simulink library "lagrange"  (R2023a)
settings: Solver=VariableStepAuto  StartTime=0.0  StopTime=10.0  RelTol=1e-3
undefined symbols (not defined in the file): b, d, g, J1, J2, J3, L, m
settings Model: Creator=Alex  LastModifiedBy=Alex

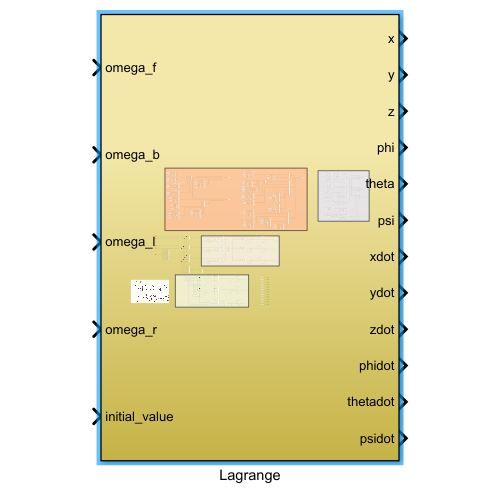
[thumbnail: Simulink's stored preview of the top-level diagram]
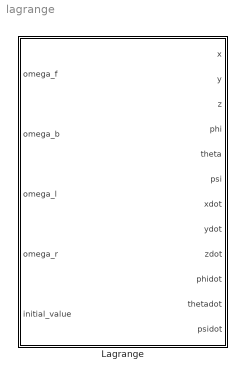
== system lagrange ==
  Lagrange : Subsystem

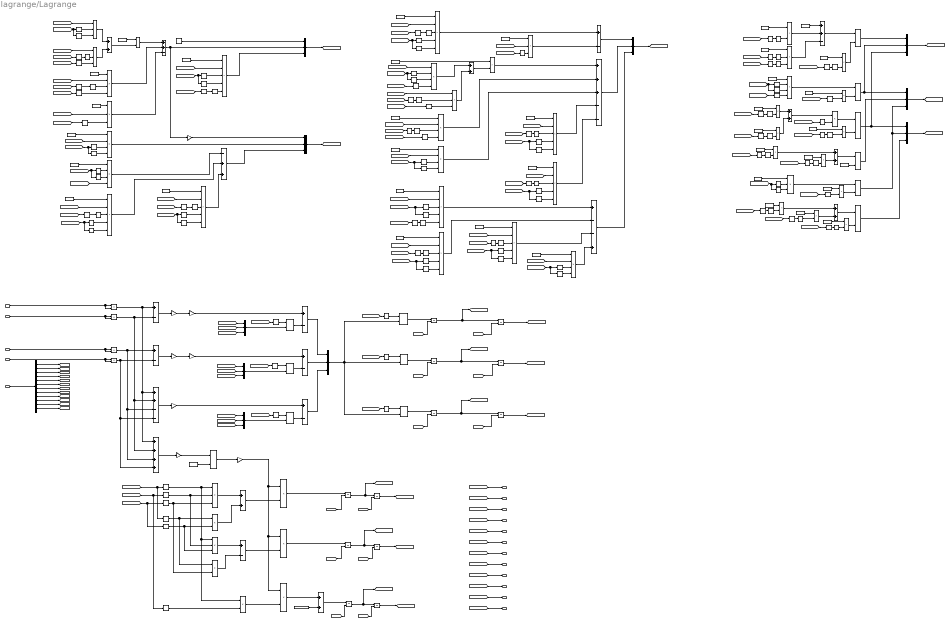
== system lagrange/Lagrange ==
  note: Rotational dynamics
  note: Matrix J^(-1) computation
  note: matrix C computation
  note: Translational dynamics
  omega_f : Inport
  omega_b : Inport  Port=2
  omega_l : Inport  Port=3
  omega_r : Inport  Port=4
  initial_value : Inport  Port=5
  Add{,1,8,11,14..16} (7 alike) : Sum  Inputs=+-
  Add{3,5,10,12,18..20} (7 alike) : Sum
  Add13 : Sum  Inputs=+--+
  Add17 : Sum  Inputs=++-
  Add2 : Sum  Inputs=++--
  Add4 : Sum  Inputs=++-
  Add6 : Sum  Inputs=++++
  Add7 : Sum  Inputs=-++
  Add9 : Sum  Inputs=+++--
  Constant : Constant  Value=0
  Constant{1,11,14,18} (4 alike) : Constant  Value=J2-J3
  Constant{10,17,20,30,33,38} (6 alike) : Constant  Value=J3
  Constant{4,8,12,15,21} (5 alike) : Constant  Value=J1
  Constant{2,5,7,13} (4 alike) : Constant  Value=J3-J2
  Constant{9,16,19,29,32,37} (6 alike) : Constant  Value=J2
  Constant{22,26,28,31,34,36} (6 alike) : Constant  Value=J2*J3
  Constant23 : Constant  Value=(J1-J3)*J2
  Constant24 : Constant  Value=(J2-J3)*J1
  Constant25 : Constant  Value=J1*J2*J3
  Constant27 : Constant  Value=-(J2-J3)
  Constant3 : Constant  Value=g
  Constant35 : Constant  Value=-(J2-J3)
  Constant6 : Constant  Value=m
  Cos{,1..7,9..10,12,15,17..18,20..21,23..24,28..30,32,34,36,38,40..41,44..45,47,49,53..55,58,60,63..64,66..67,69} (41 alike) : Trigonometry  Operator=cos
  Cos{8,11,13..14,16,19,22,25..27,31,33,35,37,39,42..43,46,48,50..52,56..57,59,61..62,65,68} (29 alike) : Trigonometry
  Demux : Demux  Outputs=12
  Divide{,1..6} (7 alike) : Product  Inputs=*/
  Gain : Gain  Gain=b
  Gain1 : Gain  Gain=L
  Gain2 : Gain  Gain=b
  Gain3 : Gain  Gain=L
  Gain4 : Gain  Gain=d
  Gain5 : Gain  Gain=b
  Gain6 : Gain  Gain=-1
  Gain7 : Gain  Gain=-1
  Integrator{,1..11} (12 alike) : Integrator  InitialConditionSource=external
  Matrix Multiply{1..6} (6 alike) : Product  Multiplication=Matrix(*)
  Mux{,1..9} (10 alike) : Mux  Inputs=3
  Product{,1..4,14,16..20,24,35,37..38,40..46,48..50} (25 alike) : Product
  Product{7,10..11,25,27..28,34,39} (8 alike) : Product  Inputs=4
  Product{9,12,21..22,29..33} (9 alike) : Product  Inputs=5
  Product{5..6,8,13,15,23,26,36,47} (9 alike) : Product  Inputs=3
  Sin{,1,8..10} (5 alike) : Trigonometry
  Sin11 : Trigonometry  Operator=cos
  Square{,1..24} (25 alike) : Math  Operator=square
  Transpose{,1..5} (6 alike) : Math  Operator=transpose
  x : Outport
  y : Outport  Port=2
  z : Outport  Port=3
  phi : Outport  Port=4
  theta : Outport  Port=5
  psi : Outport  Port=6
  xdot : Outport  Port=7
  ydot : Outport  Port=8
  zdot : Outport  Port=9
  phidot : Outport  Port=10
  thetadot : Outport  Port=11
  psidot : Outport  Port=12
  wires:
  [z] -> z/1
  [phi] -> phi/1
  [theta] -> theta/1
  [psi] -> psi/1
  [xdot] -> xdot/1
  [ydot] -> ydot/1
  [zdot] -> zdot/1
  [phidot] -> phidot/1
  [thetadot] -> thetadot/1
  [psidot] -> psidot/1
  [y] -> y/1
  [x] -> x/1
  Add10/1 -> Product18/2
  Add11/1 -> Product19/2
  Product17/1 -> Product20/2
  Sin11/1 -> Product17/2
  Product16/1 -> Add11/2
  Product15/1 -> Add11/1
  Product14/1 -> Add10/2
  Product13/1 -> Add10/1
  Sin10/1 -> Product14/2, Product15/3
  Sin9/1 -> Product14/1, Product16/1
  Cos1/1 -> Product13/3, Product16/2
  [psi] -> Sin10/1, Cos1/1
  Sin8/1 -> Product13/2, Product15/2
  [theta] -> Sin8/1, Sin11/1
  Cos/1 -> Product13/1, Product15/1, Product17/1
  [phi] -> Cos/1, Sin9/1
  Divide5/1 -> Gain7/1
  Constant6/1 -> Divide5/2
  Gain5/1 -> Divide5/1  "Fa"
  Add6/1 -> Gain5/1
  Gain4/1 -> Add16/1  "M3"
  Add2/1 -> Gain4/1
  omega_f/1 -> Product2/1, Product2/2
  omega_b/1 -> Product3/1, Product3/2
  Product2/1 -> Add1/1, Add2/3, Add6/3
  Product3/1 -> Add1/2, Add6/4, Add2/4
  Add1/1 -> Gain2/1
  Gain2/1 -> Gain3/1
  Gain3/1 -> Add15/1  "M2"
  Gain1/1 -> Add14/1  "M1"
  Gain/1 -> Gain1/1
  Add/1 -> Gain/1
  Product1/1 -> Add/2, Add6/2, Add2/2
  Product/1 -> Add/1, Add6/1, Add2/1
  omega_r/1 -> Product1/2, Product1/1
  omega_l/1 -> Product/2, Product/1
  Product20/1 -> Add3/1
  Constant3/1 -> Add3/2
  Product18/1 -> Integrator/1
  Product19/1 -> Integrator1/1
  Add3/1 -> Integrator2/1
  Integrator2/1 -> [zdot], Integrator6/1
  Integrator1/1 -> [ydot], Integrator7/1
  Integrator/1 -> [xdot], Integrator8/1
  Integrator8/1 -> [x]
  Integrator7/1 -> [y]
  Integrator6/1 -> [z]
  Integrator3/1 -> [phi]
  Integrator4/1 -> [theta]
  Integrator5/1 -> [psi]
  Integrator9/1 -> [phidot], Integrator3/1
  Integrator10/1 -> [thetadot], Integrator4/1
  Integrator11/1 -> [psidot], Integrator5/1
  Constant/1 -> Mux/1
  Constant1/1 -> Product4/1
  [thetadot] -> Product5/1
  Product4/1 -> Add4/1
  Product5/1 -> Add5/1
  [phi] -> Sin/1, Cos2/1
  Cos2/1 -> Product5/2
  Sin/1 -> Product5/3
  [psidot] -> Product6/1
  [phi] -> Sin1/1
  Sin1/1 -> Square/1
  Square/1 -> Product6/2
  [theta] -> Cos3/1
  Cos3/1 -> Product6/3
  Product6/1 -> Add5/2
  Add5/1 -> Product4/2
  Constant2/1 -> Product7/1
  Add4/1 -> Gain6/1, Mux/2
  [psidot] -> Product7/2
  [phi] -> Cos4/1
  Cos4/1 -> Square1/1
  Square1/1 -> Product7/3
  [theta] -> Cos5/1
  Cos5/1 -> Product7/4
  Product7/1 -> Add4/2
  Constant4/1 -> Product8/1
  [psidot] -> Product8/2
  [theta] -> Cos6/1
  Cos6/1 -> Product8/3
  Product8/1 -> Add4/3
  Product9/1 -> Mux/3
  Constant5/1 -> Product9/1
  [psidot] -> Product9/2
  [phi] -> Cos8/1, Cos7/1
  Cos7/1 -> Product9/3
  Cos8/1 -> Product9/4
  [theta] -> Cos9/1
  Cos9/1 -> Square2/1
  Square2/1 -> Product9/5
  Gain6/1 -> Mux1/1
  Constant7/1 -> Product10/1
  [phidot] -> Product10/2
  [phi] -> Cos11/1, Cos10/1
  Cos10/1 -> Product10/3
  Cos11/1 -> Product10/4
  Product10/1 -> Mux1/2
  Add7/1 -> Mux1/3
  Constant8/1 -> Product11/1
  [theta] -> Cos12/1, Cos13/1
  Cos13/1 -> Product11/2
  Cos12/1 -> Product11/3
  Product11/1 -> Add7/1
  [psidot] -> Product12/2
  Constant9/1 -> Product12/1
  [phi] -> Cos14/1
  Cos14/1 -> Square3/1
  Square3/1 -> Product12/3
  [theta] -> Cos16/1, Cos15/1
  Cos16/1 -> Product12/4
  Cos15/1 -> Product12/5
  Product12/1 -> Add7/2
  Constant10/1 -> Product21/1
  Product21/1 -> Add7/3
  [psidot] -> Product21/2
  Cos17/1 -> Square4/1
  [phi] -> Cos17/1
  Square4/1 -> Product21/3
  Cos18/1 -> Product21/5
  Cos19/1 -> Product21/4
  [theta] -> Cos18/1, Cos19/1
  Add8/1 -> Mux3/1
  Constant11/1 -> Product22/1
  [psidot] -> Product22/2
  [theta] -> Cos20/1
  Cos20/1 -> Square5/1
  Square5/1 -> Product22/3
  [phi] -> Cos22/1, Cos21/1
  Cos22/1 -> Product22/4
  Cos21/1 -> Product22/5
  Product22/1 -> Add8/1
  Product23/1 -> Add8/2
  Constant12/1 -> Product23/1
  [thetadot] -> Product23/2
  Cos23/1 -> Product23/3
  [theta] -> Cos23/1
  Add9/1 -> Mux3/2
  Product24/1 -> Add9/1
  Constant13/1 -> Product24/1
  Add12/1 -> Product24/2
  Product26/1 -> Add12/2
  Product25/1 -> Add12/1
  [thetadot] -> Product25/1
  Cos25/1 -> Product25/2
  [phi] -> Cos24/1, Cos25/1
  Cos24/1 -> Product25/3
  [theta] -> Cos26/1
  Cos26/1 -> Product25/4
  [phidot] -> Product26/1
  [phi] -> Cos27/1
  Cos27/1 -> Square6/1
  Square6/1 -> Product26/2
  [theta] -> Cos28/1
  Cos28/1 -> Product26/3
  Product27/1 -> Add9/2
  Product28/1 -> Add9/3
  Constant14/1 -> Product27/1
  [phidot] -> Product27/2
  Cos29/1 -> Square7/1
  [phi] -> Cos29/1
  Square7/1 -> Product27/3
  [theta] -> Cos30/1
  Cos30/1 -> Product27/4
  Constant15/1 -> Product28/1
  [psidot] -> Product28/2
  Cos31/1 -> Product28/3
  Cos32/1 -> Product28/4
  [theta] -> Cos32/1, Cos31/1
  Product29/1 -> Add9/4
  Product30/1 -> Add9/5
  Constant16/1 -> Product29/1
  Constant17/1 -> Product30/1
  [psidot] -> Product29/2
  [psidot] -> Product30/2
  Square8/1 -> Product29/3
  [phi] -> Cos33/1
  Cos33/1 -> Square8/1
  Square9/1 -> Product30/3
  [phi] -> Cos34/1
  Cos34/1 -> Square9/1
  [theta] -> Cos36/1, Cos35/1
  Cos36/1 -> Product29/5
  Cos35/1 -> Product29/4
  [theta] -> Cos37/1, Cos38/1
  Cos37/1 -> Product30/4
  Cos38/1 -> Product30/5
  Add13/1 -> Mux3/3
  Product31/1 -> Add13/1
  Product32/1 -> Add13/2
  Product33/1 -> Add13/3
  Product34/1 -> Add13/4
  Constant18/1 -> Product31/1
  [phidot] -> Product31/2
  Cos40/1 -> Product31/4
  Cos39/1 -> Product31/3
  [phi] -> Cos39/1, Cos40/1
  Cos41/1 -> Square10/1
  [theta] -> Cos41/1
  Square10/1 -> Product31/5
  Constant19/1 -> Product32/1
  [thetadot] -> Product32/2
  Cos42/1 -> Square11/1
  Square11/1 -> Product32/3
  [phi] -> Cos42/1
  [theta] -> Cos44/1, Cos43/1
  Cos44/1 -> Product32/5
  Cos43/1 -> Product32/4
  Constant20/1 -> Product33/1
  [thetadot] -> Product33/2
  Cos45/1 -> Square12/1
  [phi] -> Cos45/1
  Square12/1 -> Product33/3
  [theta] -> Cos47/1, Cos46/1
  Cos47/1 -> Product33/5
  Cos46/1 -> Product33/4
  Constant21/1 -> Product34/1
  [thetadot] -> Product34/2
  [theta] -> Cos49/1, Cos48/1
  Cos49/1 -> Product34/4
  Cos48/1 -> Product34/3
  Mux5/1 -> Matrix Multiply2/2
  [phidot] -> Mux5/1
  [thetadot] -> Mux5/2
  [psidot] -> Mux5/3
  Matrix Multiply3/1 -> Integrator10/1
  Matrix Multiply4/1 -> Integrator9/1
  Matrix Multiply5/1 -> Integrator11/1
  Mux/1 -> [c1]
  Mux1/1 -> [c2]
  Mux3/1 -> [c3]
  [c1] -> Transpose/1
  Matrix Multiply2/1 -> Add14/2
  Matrix Multiply6/1 -> Add15/2
  [c2] -> Transpose1/1
  [psidot] -> Mux2/3
  [thetadot] -> Mux2/2
  [phidot] -> Mux2/1
  Mux2/1 -> Matrix Multiply6/2
  Mux4/1 -> Matrix Multiply1/2
  [phidot] -> Mux4/1
  [thetadot] -> Mux4/2
  [psidot] -> Mux4/3
  [c3] -> Transpose2/1
  Matrix Multiply1/1 -> Add16/2
  Add15/1 -> Mux6/2
  Add14/1 -> Mux6/1
  Add16/1 -> Mux6/3
  Mux6/1 -> Matrix Multiply5/2, Matrix Multiply3/2, Matrix Multiply4/2
  Transpose/1 -> Matrix Multiply2/1
  Transpose1/1 -> Matrix Multiply6/1
  Transpose2/1 -> Matrix Multiply1/1
  Add17/1 -> Divide/1
  Constant22/1 -> Add17/1
  Product35/1 -> Add17/2
  Constant23/1 -> Product35/1
  [theta] -> Cos50/1
  Cos50/1 -> Square13/1
  Square13/1 -> Product35/2
  Constant24/1 -> Product36/1
  Product36/1 -> Add17/3
  Cos51/1 -> Square14/1
  [phi] -> Cos51/1
  Square14/1 -> Product36/2
  [theta] -> Cos52/1
  Cos52/1 -> Square15/1
  Square15/1 -> Product36/3
  Product37/1 -> Divide/2
  Constant25/1 -> Product37/1
  Cos53/1 -> Square16/1
  [theta] -> Cos53/1
  Square16/1 -> Product37/2
  Divide/1 -> Mux7/1
  Constant26/1 -> Product38/1
  Product38/1 -> Divide1/2
  Divide1/1 -> Mux8/1, Mux7/2
  [theta] -> Cos54/1
  Cos54/1 -> Product38/2
  Constant27/1 -> Product39/1
  [phi] -> Cos56/1, Cos55/1
  Cos55/1 -> Product39/2
  Cos56/1 -> Product39/3
  Cos57/1 -> Product39/4
  [theta] -> Cos57/1
  Product39/1 -> Divide1/1
  Product40/1 -> Divide2/2
  Divide2/1 -> Mux9/1, Mux7/3
  Constant28/1 -> Product40/1
  [theta] -> Cos58/1
  Cos58/1 -> Square17/1
  Square17/1 -> Product40/2
  Product41/1 -> Divide2/1
  [theta] -> Cos59/1
  Cos59/1 -> Product41/2
  Add18/1 -> Product41/1
  Product42/1 -> Add18/2
  Product43/1 -> Add18/1
  Constant29/1 -> Product43/1
  Constant30/1 -> Product42/1
  Cos60/1 -> Square18/1
  Square18/1 -> Product43/2
  [phi] -> Cos60/1
  Constant31/1 -> Divide3/2
  Add19/1 -> Divide3/1
  [phi] -> Cos61/1
  Cos61/1 -> Square19/1
  Square19/1 -> Product42/2
  Product45/1 -> Add19/1
  Product44/1 -> Add19/2
  Constant32/1 -> Product45/1
  Constant33/1 -> Product44/1
  Cos62/1 -> Square20/1
  [phi] -> Cos62/1
  Square20/1 -> Product45/2
  Square21/1 -> Product44/2
  [phi] -> Cos63/1
  Cos63/1 -> Square21/1
  Divide3/1 -> Mux8/2
  Product46/1 -> Divide4/2
  Divide4/1 -> Mux9/2, Mux8/3
  Constant34/1 -> Product46/1
  [theta] -> Cos64/1
  Cos64/1 -> Product46/2
  Product47/1 -> Divide4/1
  Constant35/1 -> Product47/1
  [phi] -> Cos66/1, Cos65/1
  Cos65/1 -> Product47/2
  Cos66/1 -> Product47/3
  Product48/1 -> Divide6/2
  Constant36/1 -> Product48/1
  Cos67/1 -> Square22/1
  [theta] -> Cos67/1
  Square22/1 -> Product48/2
  Divide6/1 -> Mux9/3
  Add20/1 -> Divide6/1
  Product50/1 -> Add20/2
  Product49/1 -> Add20/1
  Constant37/1 -> Product49/1
  [phi] -> Cos68/1
  Cos68/1 -> Square23/1
  Cos69/1 -> Square24/1
  [phi] -> Cos69/1
  Square24/1 -> Product49/2
  Square23/1 -> Product50/2
  Constant38/1 -> Product50/1
  Mux7/1 -> [inv_j1]
  Mux8/1 -> [inv_j2]
  Mux9/1 -> [inv_j3]
  Transpose3/1 -> Matrix Multiply4/1
  [inv_j1] -> Transpose3/1
  [inv_j2] -> Transpose4/1
  Transpose4/1 -> Matrix Multiply3/1
  [inv_j3] -> Transpose5/1
  Transpose5/1 -> Matrix Multiply5/1
  Gain7/1 -> Product18/1, Product19/1, Product20/1
  [psidot] -> Product11/4
  Demux/4 -> [phi0]
  Demux/3 -> [z0]
  Demux/2 -> [y0]
  Demux/6 -> [psi0]
  initial_value/1 -> Demux/1
  Demux/12 -> [psidot0]
  Demux/5 -> [theta0]
  Demux/9 -> [zdot0]
  Demux/11 -> [thetadot0]
  Demux/10 -> [phidot0]
  Demux/7 -> [xdot0]
  Demux/8 -> [ydot0]
  Demux/1 -> [x0]
  [xdot0] -> Integrator/2
  [x0] -> Integrator8/2
  [ydot0] -> Integrator1/2
  [y0] -> Integrator7/2
  [zdot0] -> Integrator2/2
  [z0] -> Integrator6/2
  [phidot0] -> Integrator9/2
  [phi0] -> Integrator3/2
  [thetadot0] -> Integrator10/2
  [theta0] -> Integrator4/2
  [psidot0] -> Integrator11/2
  [psi0] -> Integrator5/2
